simulink subsystem "ESS"  (R2021b)
settings: Solver=VariableStepAuto  StartTime=0.0  StopTime=10.0  RelTol=1e-3
model mask{ess=ess}
  mask prompts: ess "ESS data structure:"
libraries: simulink x1
settings Model: Creator=Derek  LastModifiedBy=Derek

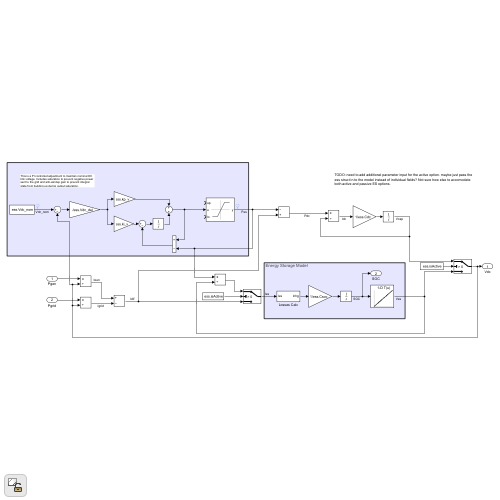
[thumbnail: Simulink's stored preview of the top-level diagram]
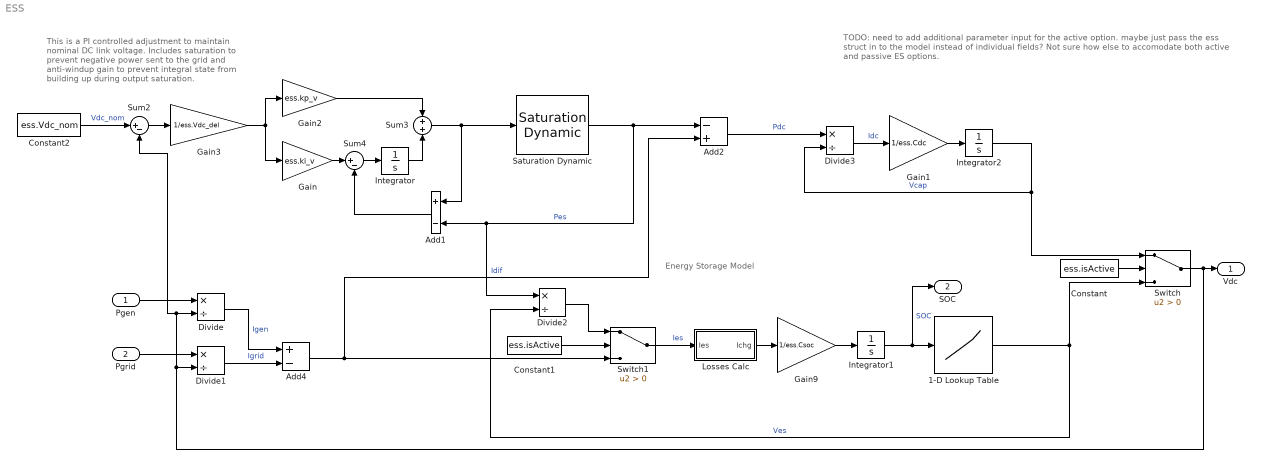
== system ESS ==
  note: TODO: need to add additional parameter input for the active option. maybe just pass the ess struct in to the model instead of individual fields? Not sure how else to accomodate both active and passive ES options.
  note: Energy Storage Model
  note: This is a PI controlled adjustment to maintain nominal DC link voltage. Includes saturation to prevent negative power sent to the grid and anti-windup gain to prevent integral state from building up during output saturation.
  Pgen : Inport
  Pgrid : Inport  Port=2
  1-D Lookup Table : Lookup_n-D  NumberOfTableDimensions=1  BreakpointsForDimension1=ess.SOC_LUT  Table=ess.Voc_LUT  InternalRulePriority=Speed  RndMeth=Simplest  InputSameDT=on
  Add1 : Sum  Inputs=+-
  Add2 : Sum  Inputs=-+
  Add4 : Sum  Inputs=+-
  Constant : Constant  Value=ess.isActive
  Constant1 : Constant  Value=ess.isActive
  Constant2 : Constant  Value=ess.Vdc_nom
  Divide{,1..3} (4 alike) : Product  Inputs=*/
  Gain : Gain  Gain=ess.ki_v
  Gain1 : Gain  Gain=1/ess.Cdc
  Gain2 : Gain  Gain=ess.kp_v
  Gain3 : Gain  Gain=1/ess.Vdc_del
  Gain9 : Gain  Gain=1/ess.Csoc
  Integrator : Integrator
  Integrator1 : Integrator  InitialCondition=ess.SOC_0
  Integrator2 : Integrator  InitialCondition=ess.Vdc_0
  Losses Calc : Subsystem
  Saturation Dynamic : simulink/Discontinuities/Saturation Dynamic  OutMin=[]  OutMax=[]  OutDataTypeStr=Inherit: Same as second input  OutDataType=fixdt(1, 16)  OutScaling=2^-10  DoSatur=off
  Sum2 : Sum  Inputs=|+-
  Sum3 : Sum
  Sum4 : Sum  Inputs=|+-
  Switch : Switch  Criteria=u2 > Threshold
  Switch1 : Switch  Criteria=u2 > Threshold
  Vdc : Outport
  SOC : Outport  Port=2
  wires:
  Pgrid/1 -> Divide1/1
  Pgen/1 -> Divide/1
  Divide1/1 -> Add4/2  "Igrid"
  Gain9/1 -> Integrator1/1
  Divide/1 -> Add4/1  "Igen"
  Integrator1/1 -> 1-D Lookup Table/1, SOC/1  "SOC"
  Switch1/1 -> Losses Calc/1(Ies)  "Ies"
  Losses Calc/1(Ichg) -> Gain9/1
  Switch/1 -> Vdc/1, Divide1/2, Divide/2, Sum2/2
  Gain1/1 -> Integrator2/1
  Divide3/1 -> Gain1/1  "Idc"
  Constant/1 -> Switch/2
  Integrator2/1 -> Divide3/2, Switch/1  "Vcap"
  1-D Lookup Table/1 -> Switch/3, Divide2/2  "Ves"
  Constant1/1 -> Switch1/2
  Add4/1 -> Switch1/3, Add2/2  "Idif"
  Gain/1 -> Sum4/1
  Add1/1 -> Sum4/2
  Integrator/1 -> Sum3/2
  Sum4/1 -> Integrator/1
  Saturation Dynamic/1 -> Add2/1, Add1/2, Divide2/1  "Pes"
  Gain3/1 -> Gain/1, Gain2/1
  Gain2/1 -> Sum3/1
  Sum2/1 -> Gain3/1
  Sum3/1 -> Saturation Dynamic/2, Add1/1
  Constant2/1 -> Sum2/1  "Vdc_nom"
  Divide2/1 -> Switch1/1
  Add2/1 -> Divide3/1  "Pdc"

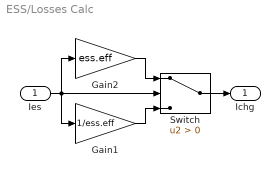
== system ESS/Losses Calc ==
  Ies : Inport
  Gain1 : Gain  Gain=1/ess.eff
  Gain2 : Gain  Gain=ess.eff
  Switch : Switch  Criteria=u2 > Threshold
  Ichg : Outport
  wires:
  Gain1/1 -> Switch/3
  Gain2/1 -> Switch/1
  Switch/1 -> Ichg/1
  Ies/1 -> Switch/2, Gain2/1, Gain1/1
